simulink model "erreurVi"  (R2017b)
settings: Solver=VariableStepAuto  StartTime=0.0  StopTime=2000  RelTol=1e-3
values from neighbouring files (symbols this model uses):
  Dev = Kp_ev.den{1}    [final2016.m]    (also in ordretwo.m)
  DPro = tfd3.den{1}    [final2016.m]    (also in ordretwo.m)
  Nev = Kp_ev.num{1}    [final2016.m]    (also in ordretwo.m)
  NPro = tfd3.num{1}    [final2016.m]    (also in ordretwo.m)
  te2 = 60    [final2016.m]    (also in ordretwo.m = 2.5)
libraries: simulink x1
settings Model: Creator=lencs  LastModifiedBy=lencs

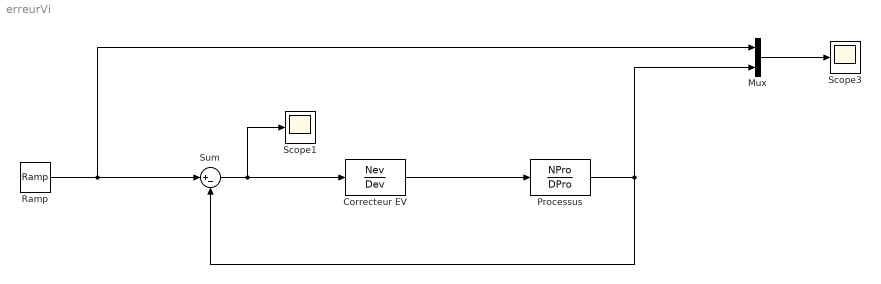
== system erreurVi ==
  Correcteur EV : DiscreteFilter  Numerator=Nev  Denominator=Dev  SampleTime=te2
  Mux : Mux  Inputs=2
  Processus : DiscreteFilter  Numerator=NPro  Denominator=DPro  SampleTime=te2
  Ramp : simulink/Sources/Ramp  slope=1  start=0  X0=0
  Scope1 : Scope
  Scope3 : Scope
  Sum : Sum  Inputs=|+-
  wires:
  Ramp/1 -> Mux/1, Sum/1
  Correcteur EV/1 -> Processus/1
  Sum/1 -> Scope1/1, Correcteur EV/1
  Processus/1 -> Sum/2, Mux/2
  Mux/1 -> Scope3/1
